simulink model "MotorCtrl_FOC_Physic"  (R2023b)
settings: Solver=FixedStepDiscrete  StartTime=0.0  StopTime=10  FixedStep=MC_Sim_BaseStep  RelTol=1e-3  EnableMultiTasking=on
values from neighbouring files (symbols this model uses):
  MC_MOS_DeadTime = 1.0E-6    [MotorControlDataDictionary_Math.sldd]    (also in MotorControlDataDictionary_Physic.sldd)
  MC_Motor_Mechinal_Inertia = 0.0103    [MotorControlDataDictionary_Math.sldd]    (also in MotorControlDataDictionary_Physic.sldd)
  MC_Motor_Phi = 0.0059190254913385806    [MotorControlDataDictionary_Math.sldd]    (also in MotorControlDataDictionary_Physic.sldd)
  MC_Motor_Rotor_Pn = 4.0    [MotorControlDataDictionary_Math.sldd]    (also in MotorControlDataDictionary_Physic.sldd)
  MC_Motor_Stator_Ld = 5.6345E-5    [MotorControlDataDictionary_Math.sldd]    (also in MotorControlDataDictionary_Physic.sldd)
  MC_Motor_Stator_Lq = 5.6345E-5    [MotorControlDataDictionary_Math.sldd]    (also in MotorControlDataDictionary_Physic.sldd)
  MC_Motor_Stator_Rs = 0.0286    [MotorControlDataDictionary_Math.sldd]    (also in MotorControlDataDictionary_Physic.sldd)
  MC_Param_CurrentPI_Ki = 0.0071879639914134473    [MotorControlDataDictionary_Math.sldd]    (also in MotorControlDataDictionary_Physic.sldd)
  MC_Param_CurrentPI_Kp = 0.283220860906427    [MotorControlDataDictionary_Math.sldd]    (also in MotorControlDataDictionary_Physic.sldd)
  MC_Param_CurrentPI_UdInteMax = 7.794228634059948    [MotorControlDataDictionary_Math.sldd]    (also in MotorControlDataDictionary_Physic.sldd)
  MC_Param_CurrentPI_UdInteMin = -7.794228634059948    [MotorControlDataDictionary_Math.sldd]    (also in MotorControlDataDictionary_Physic.sldd)
  MC_Param_CurrentPI_UdMax = 7.794228634059948    [MotorControlDataDictionary_Math.sldd]    (also in MotorControlDataDictionary_Physic.sldd)
  MC_Param_CurrentPI_UdMin = -7.794228634059948    [MotorControlDataDictionary_Math.sldd]    (also in MotorControlDataDictionary_Physic.sldd)
  MC_Param_CurrentPI_UqInteMax = 7.794228634059948    [MotorControlDataDictionary_Math.sldd]    (also in MotorControlDataDictionary_Physic.sldd)
  MC_Param_CurrentPI_UqInteMin = -7.794228634059948    [MotorControlDataDictionary_Math.sldd]    (also in MotorControlDataDictionary_Physic.sldd)
  MC_Param_CurrentPI_UqMax = 7.794228634059948    [MotorControlDataDictionary_Math.sldd]    (also in MotorControlDataDictionary_Physic.sldd)
  MC_Param_CurrentPI_UqMin = -7.794228634059948    [MotorControlDataDictionary_Math.sldd]    (also in MotorControlDataDictionary_Physic.sldd)
  MC_Param_Flux_Gamma = 750000.0    [MotorControlDataDictionary_Math.sldd]    (also in MotorControlDataDictionary_Physic.sldd)
  MC_Param_PhasetoReal = 500.0    [MotorControlDataDictionary_Math.sldd]    (also in MotorControlDataDictionary_Physic.sldd)
  MC_Param_SMO_CoffA = 0.97462064069571386    [MotorControlDataDictionary_Math.sldd]    (also in MotorControlDataDictionary_Physic.sldd)
  MC_Param_SMO_CoffB = 0.88739018546454884    [MotorControlDataDictionary_Math.sldd]    (also in MotorControlDataDictionary_Physic.sldd)
  MC_Param_SpeedCtrl_IdMax = 60.0    [MotorControlDataDictionary_Math.sldd]    (also in MotorControlDataDictionary_Physic.sldd)
  MC_Param_SpeedCtrl_IdMin = -60.0    [MotorControlDataDictionary_Math.sldd]    (also in MotorControlDataDictionary_Physic.sldd)
  MC_Param_SpeedCtrl_IqMax = 60.0    [MotorControlDataDictionary_Math.sldd]    (also in MotorControlDataDictionary_Physic.sldd)
  MC_Param_SpeedCtrl_IqMin = -60.0    [MotorControlDataDictionary_Math.sldd]    (also in MotorControlDataDictionary_Physic.sldd)
  MC_Param_SpeedPI_Ki = 0.57248683633241571    [MotorControlDataDictionary_Math.sldd]    (also in MotorControlDataDictionary_Physic.sldd)
  MC_Param_SpeedPI_Kp = 9.1114109857344836    [MotorControlDataDictionary_Math.sldd]    (also in MotorControlDataDictionary_Physic.sldd)
  MC_Param_SpeedtoTheta = 5.0E-5    [MotorControlDataDictionary_Math.sldd]    (also in MotorControlDataDictionary_Physic.sldd)
  MC_Param_SVPWM_DutyMax = 0.98    [MotorControlDataDictionary_Math.sldd]    (also in MotorControlDataDictionary_Physic.sldd)
  MC_Param_SVPWM_DutyMin = 0.02    [MotorControlDataDictionary_Math.sldd]    (also in MotorControlDataDictionary_Physic.sldd)
  MC_Param_SVPWM_SampleOffset1 = 0.02    [MotorControlDataDictionary_Math.sldd]    (also in MotorControlDataDictionary_Physic.sldd)
  MC_Param_SVPWM_SampleOffset2 = 0.015    [MotorControlDataDictionary_Math.sldd]    (also in MotorControlDataDictionary_Physic.sldd)
  MC_Param_SVPWM_SampleValid = 0.011999999999999999    [MotorControlDataDictionary_Math.sldd]    (also in MotorControlDataDictionary_Physic.sldd)
  MC_Sample_CurrentNoise = 1.0E-15    [MotorControlDataDictionary_Math.sldd]    (also in MotorControlDataDictionary_Physic.sldd)
  MC_Sample_VbusNoise = 1.0E-15    [MotorControlDataDictionary_Math.sldd]    (also in MotorControlDataDictionary_Physic.sldd)
  MC_Sim_BaseStep = 5.0E-8    [MotorControlDataDictionary_Math.sldd]    (also in MotorControlDataDictionary_Physic.sldd)
  MC_Sim_HFTStep = 5.0E-5    [MotorControlDataDictionary_Math.sldd]    (also in MotorControlDataDictionary_Physic.sldd)
  MC_Sim_MFTStep = 0.002    [MotorControlDataDictionary_Math.sldd]    (also in MotorControlDataDictionary_Physic.sldd)
libraries: simulink x17, nesl_utility x15, ee_lib x10, fl_lib x8
(part 1 of 3)
settings Model: DataDictionary=MotorControlDataDictionary_Physic.sldd  SimulationMode=accelerator  Creator=YXuan  LastModifiedBy=YXuan
settings SolverCC: AutoInsertRateTranBlk=on
settings OptimizationCC: DefaultParameterBehavior=Inlined  DefaultUnderspecifiedDataType=single  EnhancedBackFolding=on  PassReuseOutputArgsAs=Individual arguments  ZeroExternalMemoryAtStartup=off  ZeroInternalMemoryAtStartup=off  EfficientFloat2IntCast=on  OptimizeBlockOrder=speed  DifferentSizesBufferReuse=on  OptimizationCustomize=off  EfficientTunableParamExpr=on
settings DebuggingCC: ParameterPrecisionLossMsg=none
settings HardwareCC: ProdBitPerPointer=32  ProdBitPerSizeT=32  ProdBitPerPtrDiffT=32  ProdLargestAtomicInteger=Long  ProdLargestAtomicFloat=Double  ProdWordSize=32  ProdHWDeviceType=ARM Compatible->ARM Cortex-M
settings ModelReferenceCC: EnableRefExpFcnMdlSchedulingChecks=on
settings SFSimCC: MATLABDynamicMemAlloc=off
settings RTWCC: Description=Embedded Coder  SystemTargetFile=ert.tlc  GenCodeOnly=on  TemplateMakefile=ert_default_tmf  Toolchain=Microsoft Visual C++ 2022 v17.0 | nmake (64-bit Windows)
settings CodeAppCC: ForceParamTrailComments=on  IgnoreCustomStorageClasses=off  IgnoreTestpoints=on  OperatorAnnotations=on  SimulinkDataObjDesc=on  SFDataObjDesc=on  InsertBlockDesc=on
settings ERTTargetCC: TargetLangStandard=C99 (ISO)  InferredTypesCompatibility=on  GenerateSampleERTMain=on  CombineSignalStateStructs=on  SupportAbsoluteTime=off  SupportNonFinite=off  SupportComplex=off  RemoveDisableFunc=on  InlinedParameterPlacement=NonHierarchical  ERTCustomFileTemplate=example_file_process.tlc

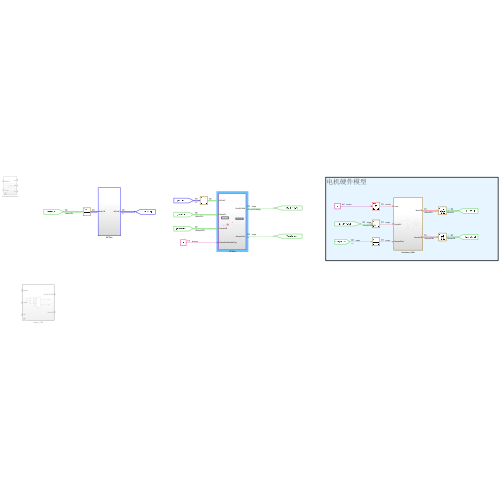
[thumbnail: Simulink's stored preview of the top-level diagram]
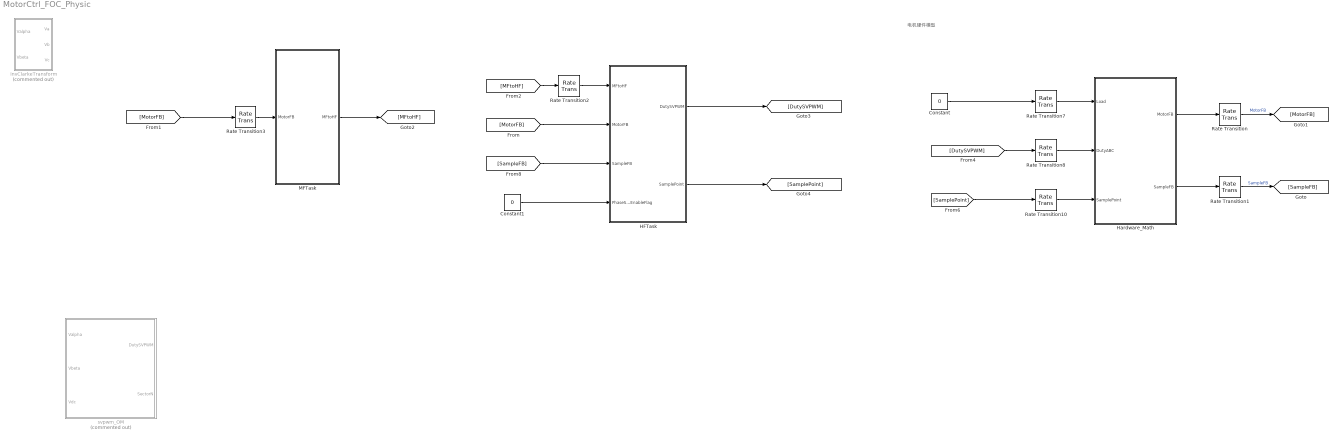
== system MotorCtrl_FOC_Physic ==
  note: 电机硬件模型
  Constant : Constant  Value=0
  Constant1 : Constant  Value=0  OutDataTypeStr=boolean
  HFTask : Subsystem  TreatAsAtomicUnit=on  SystemSampleTime=MC_Sim_HFTStep
  Hardware_Math : Subsystem  SystemSampleTime=MC_Sim_BaseStep  VariantControl=MC_Hardware_Motor_Model ==1&MC_Hardware_MotorMOS_Model==1
  MFTask : Subsystem  TreatAsAtomicUnit=on  SystemSampleTime=MC_Sim_MFTStep
  Rate Transition : RateTransition  OutPortSampleTime=MC_Sim_HFTStep
  Rate Transition1 : RateTransition  OutPortSampleTime=MC_Sim_HFTStep
  Rate Transition10 : RateTransition  OutPortSampleTime=MC_Sim_BaseStep
  Rate Transition2 : RateTransition  OutPortSampleTime=MC_Sim_HFTStep
  Rate Transition3 : RateTransition  OutPortSampleTime=MC_Sim_MFTStep
  Rate Transition7 : RateTransition  OutPortSampleTime=MC_Sim_BaseStep
  Rate Transition8 : RateTransition  OutPortSampleTime=MC_Sim_BaseStep
  invClarkeTransform : Subsystem  Commented=on
  svpwm_OM : Subsystem  Commented=on  TreatAsAtomicUnit=on  SystemSampleTime=MC_Sim_HFTStep
      settings: RTWSystemCode=Nonreusable function  RTWFcnNameOpts=Use subsystem name
  wires:
  Hardware_Math/2(SampleFB) -> Rate Transition1/1
  Rate Transition8/1 -> Hardware_Math/2(DutyABC)
  Hardware_Math/1(MotorFB) -> Rate Transition/1
  [SamplePoint] -> Rate Transition10/1
  [DutySVPWM] -> Rate Transition8/1
  Rate Transition1/1 -> [SampleFB]  "SampleFB"
  Constant/1 -> Rate Transition7/1
  Rate Transition10/1 -> Hardware_Math/3(SamplePoint)
  Rate Transition7/1 -> Hardware_Math/1(Load)
  Rate Transition/1 -> [MotorFB]  "MotorFB"
  HFTask/2(SamplePoint) -> [SamplePoint]
  Rate Transition2/1 -> HFTask/1(MFtoHF)
  [MFtoHF] -> Rate Transition2/1
  Rate Transition3/1 -> MFTask/1(MotorFB)
  Constant1/1 -> HFTask/4(PhaseShortEnableFlag)
  [MotorFB] -> Rate Transition3/1
  [SampleFB] -> HFTask/3(SampleFB)
  MFTask/1(MFtoHF) -> [MFtoHF]
  [MotorFB] -> HFTask/2(MotorFB)
  HFTask/1(DutySVPWM) -> [DutySVPWM]

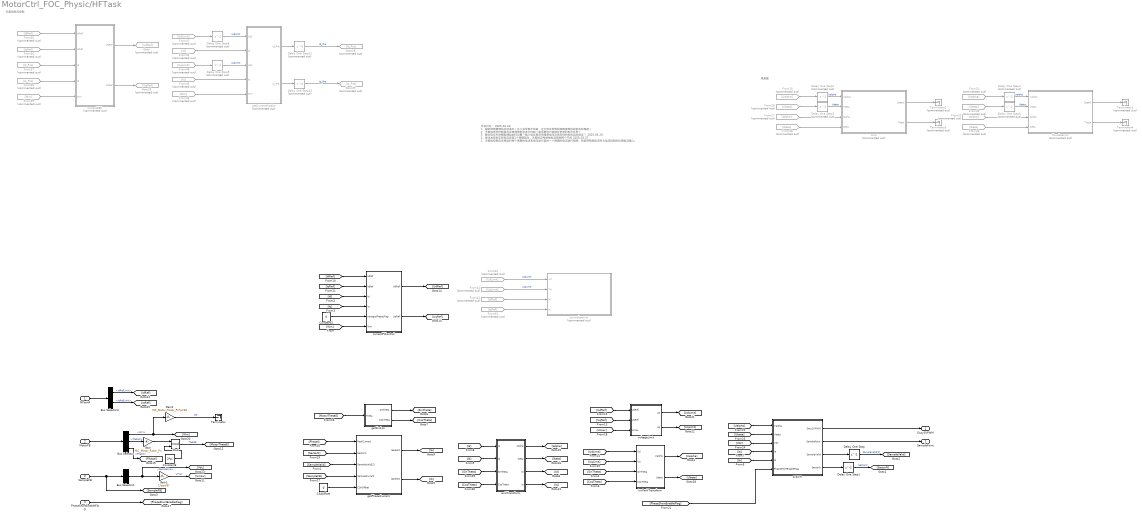
== system MotorCtrl_FOC_Physic/HFTask ==
  note: 观测器
  note: 无差拍电流控制
  note: 开发日志：
      | 2025.03.24:
      | 1、磁链观测器增益应该适中（过小会导致不收敛，过大则会导致观测角度相位超前实际角度）
      | 2、无差拍电流控制是否采用预测电流进行控制？是否要进行旋转反电势的电压补偿？
      | 3、静态电压补偿模型增益如何设置？输入电压是采用理想电压还是采样的电机实际电压？
      | 2025.03.25:
      | 1、测试发现电压和电流呈现2个周期延时，无差拍应考虑做电流预测两个节拍
      | 2025.03.27：
      | 1、无差拍控制应采用延时两个周期的电流和电压进行延时一个周期的电流进行预测，然后用预测电流作为电流控制的反馈电流输入。
  MFtoHF : Inport
  MotorFB : Inport  Port=2
  SampleFB : Inport  Port=3
  PhaseShortEnableFlag : Inport  Port=4
  Bus Selector : BusSelector  OutputSignals=Wm,ThetaM,PhaseI
  Bus Selector1 : BusSelector  OutputSignals=SampleVus
  Bus Selector3 : BusSelector  OutputSignals=IdRefLimit,IqRefLimit
  CSAOffset : Constant  Value=0  OutDataTypeStr=single
  Constant2 : Constant  Value=0  OutDataTypeStr=boolean
  Constant6 : Constant  Value=2*pi  OutDataTypeStr=single
  Delay One Step : Delay
  Delay One Step1 : Delay
  Delay One Step12 : Delay  Commented=on  DelayLength=0
  Delay One Step13 : Delay  Commented=on  DelayLength=0
  Delay One Step{2..5} (4 alike) : Delay  Commented=on
  Delay One Step8 : Delay  Commented=on  DelayLength=1
  Delay One Step9 : Delay  Commented=on  DelayLength=1
  From25 : From  Commented=on  GotoTag=Ualpha
  From26 : From  Commented=on  GotoTag=Ubeta
  From27 : From  Commented=on  GotoTag=Ialpha
  From28 : From  Commented=on  GotoTag=Ibeta
  From31 : From  Commented=on  GotoTag=Ualpha
  From32 : From  Commented=on  GotoTag=Ubeta
  From33 : From  Commented=on  GotoTag=Ialpha
  From34 : From  Commented=on  GotoTag=Ibeta
  From35 : From  Commented=on  GotoTag=IdRef
  From36 : From  Commented=on  GotoTag=IqRef
  From37 : From  Commented=on  GotoTag=Id_Pre
  From38 : From  Commented=on  GotoTag=Iq_Pre
  From39 : From  Commented=on  GotoTag=Wm
  From40 : From  Commented=on  GotoTag=UdLimit
  From41 : From  Commented=on  GotoTag=UqLimit
  From42 : From  Commented=on  GotoTag=IdRef
  From43 : From  Commented=on  GotoTag=IqRef
  From44 : From  Commented=on  GotoTag=Id
  From45 : From  Commented=on  GotoTag=Iq
  From46 : From  Commented=on  GotoTag=Wm
  From47 : From  Commented=on  GotoTag=UdLimit
  From48 : From  Commented=on  GotoTag=UqLimit
  Gain : Gain  Gain=MC_Motor_Rotor_Pn  OutDataTypeStr=single
  Gain1 : Gain  Gain=1/sqrt(3)  OutDataTypeStr=single
  Gain2 : Gain  Gain=MC_Motor_Rotor_Pn*pi/30
  Goto : Goto  Commented=on  GotoTag=UdRef
  Goto26 : Goto  Commented=on  GotoTag=UqRef
  Goto28 : Goto  Commented=on  GotoTag=Id_Pre
  Goto29 : Goto  Commented=on  GotoTag=Iq_Pre
  Mod : Math  Operator=mod
  Terminator : Terminator
  Terminator{1..4} (4 alike) : Terminator  Commented=on
  axisTransform : Subsystem
  currentDBC : Subsystem  Commented=on
  currentPIControl : Subsystem
  fluxobservor : Subsystem  Commented=on
  getCurrentPredict : Subsystem  Commented=on
  getPhaseCurrent : Subsystem
  getSinCos : Subsystem
  invParkTransform : Subsystem
  scvmobservor : Subsystem  Commented=on
  smo : Subsystem  Commented=on
  svpwm : Subsystem  TreatAsAtomicUnit=on
  voltageLimit : Subsystem
  DutySVPWM : Outport
  SamplePoint : Outport  Port=2
  wires:
  MFtoHF/1 -> Bus Selector3/1
  Delay One Step2/1 -> smo/1(Valpha)  "Ualpha"
  From25/1 -> Delay One Step2/1
  Delay One Step3/1 -> smo/2(Vbeta)  "Ubeta"
  From26/1 -> Delay One Step3/1
  From27/1 -> smo/3(Ialpha)
  From28/1 -> smo/4(Ibeta)
  smo/1(Speed) -> Terminator2/1
  smo/2(Theta) -> Terminator3/1
  [PhaseShortEnableFlag] -> svpwm/6(PhaseShortEnableFlag)
  [Umax] -> voltageLimit/3(Umax)
  svpwm/4(SectorN) -> Delay One Step1/1
  axisTransform/2(Ibeta) -> [Ibeta]
  svpwm/3(SampleValid) -> Delay One Step/1
  svpwm/1(DutySVPWM) -> DutySVPWM/1
  [SampleFB] -> getPhaseCurrent/4(SampleCurrent)
  [SectorN] -> getPhaseCurrent/2(SectorN)
  [UdRef] -> voltageLimit/1(UdRef)
  [UdLimit] -> invParkTransform/1(Ud)
  currentPIControl/1(UdRef) -> [UdRef]
  [Ubeta] -> svpwm/2(Vbeta)
  axisTransform/1(Ialpha) -> [Ialpha]
  [UqRef] -> voltageLimit/2(UqRef)
  [Ualpha] -> svpwm/1(Valpha)
  [Ia] -> axisTransform/1(Ia)
  svpwm/2(SamplePoint) -> SamplePoint/1
  currentPIControl/2(UqRef) -> [UqRef]
  [Vdc] -> svpwm/3(Vdc)
  voltageLimit/1(Ud) -> [UdLimit]
  [MotorThetaE] -> getSinCos/1(Theta)
  [Id] -> currentPIControl/3(Id)
  getSinCos/1(SinTheta) -> [SinTheta]
  [SampleValid] -> getPhaseCurrent/3(SampleValid[2])
  axisTransform/3(Id) -> [Id]
  getPhaseCurrent/2(Ibselect) -> [Ib]
  [Wm] -> currentPIControl/6(Wm)
  axisTransform/4(Iq) -> [Iq]
  [Iq] -> currentPIControl/4(Iq)
  Constant2/1 -> currentPIControl/5(IntregralResetFlag)
  [Ib] -> axisTransform/2(Ib)
  [UqLimit] -> invParkTransform/2(Uq)
  [SinTheta] -> invParkTransform/3(SinTheta)
  Delay One Step1/1 -> [SectorN]  "SectorN"
  [CosTheta] -> invParkTransform/4(CosTheta)
  [PhaseI] -> getPhaseCurrent/1(RealCurrent)
  invParkTransform/1(Ualpha) -> [Ualpha]
  Delay One Step/1 -> [SampleValid]  "SampleValid[2]"
  getSinCos/2(CosTheta) -> [CosTheta]
  voltageLimit/2(Uq) -> [UqLimit]
  [SinTheta] -> axisTransform/3(SinTheta)
  getPhaseCurrent/1(Iaselect) -> [Ia]
  CSAOffset/1 -> getPhaseCurrent/5(CSAOffset)
  [CosTheta] -> axisTransform/4(CosTheta)
  invParkTransform/2(Ubeta) -> [Ubeta]
  [Ib] -> svpwm/5(Ib)
  [Ia] -> svpwm/4(Ia)
  Bus Selector/2 -> Gain/1  "<ThetaM>"
  PhaseShortEnableFlag/1 -> [PhaseShortEnableFlag]
  Bus Selector/1 -> Gain2/1, [Wm]  "<Wm>"
  Mod/1 -> [MotorThetaE]  "ThetaE"
  Bus Selector/3 -> [PhaseI]  "<PhaseI>"
  Gain/1 -> Mod/1
  Bus Selector1/1 -> [Vdc], Gain1/1  "<SampleVus>"
  SampleFB/1 -> [SampleFB], Bus Selector1/1
  Gain1/1 -> [Umax]  "Umax"
  Constant6/1 -> Mod/2
  MotorFB/1 -> Bus Selector/1
  Bus Selector3/1 -> [IdRef]  "<IdRefLimit>"
  Bus Selector3/2 -> [IqRef]  "<IqRefLimit>"
  [IdRef] -> currentPIControl/1(IdRef)
  [IqRef] -> currentPIControl/2(IqRef)
  From34/1 -> fluxobservor/4(Ibeta)
  From33/1 -> fluxobservor/3(Ialpha)
  From32/1 -> Delay One Step5/1
  From31/1 -> Delay One Step4/1
  Delay One Step4/1 -> fluxobservor/1(Valpha)  "Ualpha"
  Delay One Step5/1 -> fluxobservor/2(Vbeta)  "Ubeta"
  fluxobservor/1(Speed) -> Terminator1/1
  fluxobservor/2(Theta) -> Terminator4/1
  currentDBC/2(UqRef) -> Goto26/1
  From36/1 -> currentDBC/2(IqRef)
  From35/1 -> currentDBC/1(IdRef)
  From37/1 -> currentDBC/3(Id)
  From38/1 -> currentDBC/4(Iq)
  From39/1 -> currentDBC/5(Wm)
  From41/1 -> scvmobservor/2(Vq)  "UqLimit"
  From40/1 -> scvmobservor/1(Vd)  "UdLimit"
  From42/1 -> scvmobservor/3(Id)
  From43/1 -> scvmobservor/4(Iq)
  Gain2/1 -> Terminator/1  "We"
  From44/1 -> getCurrentPredict/2(Id)
  From45/1 -> getCurrentPredict/4(Iq)
  From46/1 -> getCurrentPredict/5(Wm)
  From47/1 -> Delay One Step8/1
  From48/1 -> Delay One Step9/1
  getCurrentPredict/1(Id_Pre) -> Delay One Step12/1
  getCurrentPredict/2(Iq_Pre) -> Delay One Step13/1
  currentDBC/1(UdRef) -> Goto/1
  Delay One Step8/1 -> getCurrentPredict/1(Ud1)  "UdLimit"
  Delay One Step9/1 -> getCurrentPredict/3(Uq1)  "UqLimit"
  Delay One Step12/1 -> Goto28/1  "Id_Pre"
  Delay One Step13/1 -> Goto29/1  "Iq_Pre"

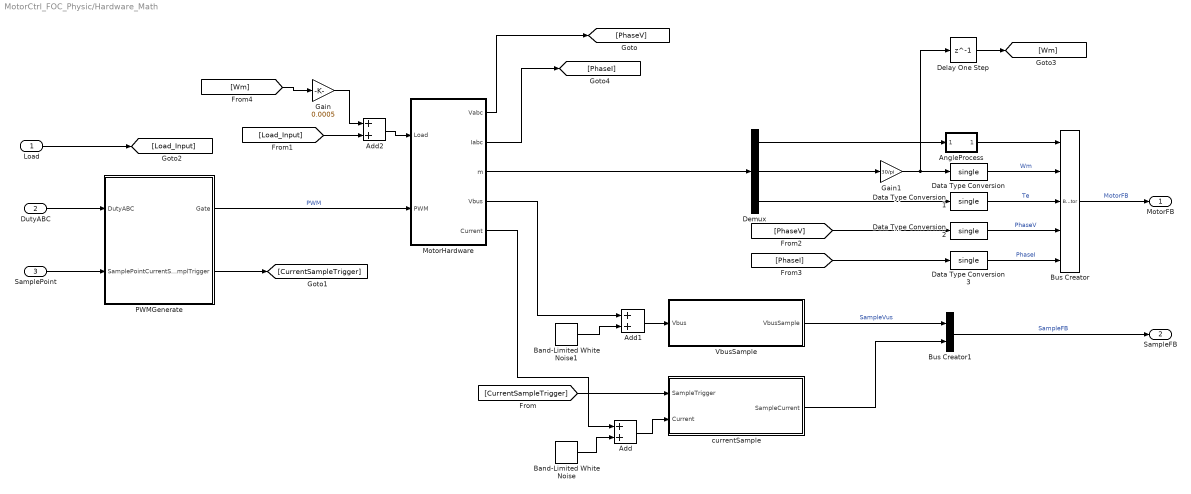
== system MotorCtrl_FOC_Physic/Hardware_Math ==
  Load : Inport
  DutyABC : Inport  Port=2
  SamplePoint : Inport  Port=3
  Add : Sum
  Add1 : Sum
  Add2 : Sum
  AngleProcess : Subsystem
  Band-Limited White Noise : simulink/Sources/Band-Limited White Noise  Cov=[MC_Sample_CurrentNoise]  Ts=MC_Sim_BaseStep  seed=[23341]
  Band-Limited White Noise1 : simulink/Sources/Band-Limited White Noise  Cov=[MC_Sample_VbusNoise]  Ts=MC_Sim_BaseStep  seed=[23341]
  Bus Creator : BusCreator  Inputs=5
  Bus Creator1 : BusCreator  Inputs=2
  Data Type Conversion{,1..3} (4 alike) : DataTypeConversion  OutDataTypeStr=single  SaturateOnIntegerOverflow=off  RndMeth=Floor
  Delay One Step : Delay  DelayLength=1
  Demux : Demux  Outputs=3
  Gain : Gain  Gain=0.0005
  Gain1 : Gain  Gain=30/pi
  MotorHardware : Subsystem
  PWMGenerate : Subsystem  SystemSampleTime=MC_Sim_BaseStep
  VbusSample : Subsystem
  currentSample : Subsystem  Variant=on  VariantControl=Subsystem
  MotorFB : Outport
  SampleFB : Outport  Port=2
  wires:
  Band-Limited White Noise/1 -> Add/2
  Add/1 -> currentSample/2(Current)
  Add1/1 -> VbusSample/1(Vbus)
  Band-Limited White Noise1/1 -> Add1/2
  [CurrentSampleTrigger] -> currentSample/1(SampleTrigger)
  PWMGenerate/2(CurrentSamplTrigger) -> [CurrentSampleTrigger]
  Demux/2 -> Gain1/1
  DutyABC/1 -> PWMGenerate/1(DutyABC)
  Demux/1 -> AngleProcess/1(In1)
  SamplePoint/1 -> PWMGenerate/2(SamplePoint)
  Demux/3 -> Data Type Conversion1/1
  Load/1 -> [Load_Input]
  Gain1/1 -> Delay One Step/1, Data Type Conversion/1
  AngleProcess/1(Out1) -> Bus Creator/1
  [PhaseV] -> Data Type Conversion2/1
  [PhaseI] -> Data Type Conversion3/1
  VbusSample/1(VbusSample) -> Bus Creator1/1  "SampleVus"
  currentSample/1(SampleCurrent) -> Bus Creator1/2
  Bus Creator1/1 -> SampleFB/1  "SampleFB"
  PWMGenerate/1(Gate) -> MotorHardware/2(PWM)  "PWM"
  MotorHardware/1(Vabc) -> [PhaseV]
  MotorHardware/2(Iabc) -> [PhaseI]
  MotorHardware/3(m) -> Demux/1
  MotorHardware/5(Current) -> Add/1
  MotorHardware/4(Vbus) -> Add1/1
  Data Type Conversion/1 -> Bus Creator/2  "Wm"
  Data Type Conversion1/1 -> Bus Creator/3  "Te"
  Data Type Conversion2/1 -> Bus Creator/4  "PhaseV"
  Data Type Conversion3/1 -> Bus Creator/5  "PhaseI"
  Bus Creator/1 -> MotorFB/1  "MotorFB"
  Add2/1 -> MotorHardware/1(Load)
  [Load_Input] -> Add2/2
  [Wm] -> Gain/1
  Gain/1 -> Add2/1
  Delay One Step/1 -> [Wm]

== system MotorCtrl_FOC_Physic/MFTask ==
  MotorFB : Inport
  Bus Creator : BusCreator  Inputs=2
  Bus Selector : BusSelector  OutputSignals=Wm
  Constant : Constant  Value=1500  OutDataTypeStr=single
  From2 : From  Commented=on  GotoTag=SpeedTarget
  From3 : From  Commented=on  GotoTag=SpeedMotor
  Goto : Goto  Commented=on  GotoTag=IdRef
  Goto1 : Goto  Commented=on  GotoTag=IqRef
  getCurrentLimit : Subsystem
  piofSpeed : Subsystem
  smcofSpeed : Subsystem  Commented=on
  MFtoHF : Outport
  wires:
  MotorFB/1 -> Bus Selector/1
  Bus Selector/1 -> [SpeedMotor]  "<Wm>"
  Bus Creator/1 -> MFtoHF/1
  smcofSpeed/1(IdRef) -> Goto/1
  smcofSpeed/2(IqRef) -> Goto1/1
  piofSpeed/1(IdRef) -> [IdRef]
  piofSpeed/2(IqRef) -> [IqRef]
  getCurrentLimit/2(IqRefLimit) -> [IqRefLimit]
  getCurrentLimit/1(IdRefLimit) -> [IdRefLimit]
  [IdRefLimit] -> Bus Creator/1
  [IqRefLimit] -> Bus Creator/2
  Constant/1 -> [SpeedTarget]  "SpeedTarget"
  From2/1 -> smcofSpeed/1(SpeedTarget)
  From3/1 -> smcofSpeed/2(SpeedReal)
  [IdRef] -> getCurrentLimit/1(IdRef)
  [IqRef] -> getCurrentLimit/2(IqRef)
  [SpeedTarget] -> piofSpeed/1(SpeedTarget)
  [SpeedMotor] -> piofSpeed/2(SpeedReal)

== system MotorCtrl_FOC_Physic/invClarkeTransform ==
  Valpha : Inport
  Vbeta : Inport  Port=2
  Add : Sum
  Gain : Gain  Gain=-1/2
  Gain1 : Gain  Gain=sqrt(3)/2
  Subtract : Sum  Inputs=+-
  Va : Outport
  Vb : Outport  Port=2
  Vc : Outport  Port=3
  wires:
  Valpha/1 -> Gain/1, Va/1  "Va"
  Vbeta/1 -> Gain1/1
  Gain/1 -> Subtract/1, Add/1
  Gain1/1 -> Subtract/2, Add/2
  Add/1 -> Vb/1  "Vb"
  Subtract/1 -> Vc/1  "Vc"

== system MotorCtrl_FOC_Physic/svpwm_OM ==
  Valpha : Inport
  Vbeta : Inport  Port=2
  Vdc : Inport  Port=3
  getVoltageExchange : Subsystem
  setDTCompelte : Subsystem
  DutySVPWM : Outport
  SectorN : Outport  Port=2
  wires:
  getVoltageExchange/4(Vmed) -> setDTCompelte/4(Vmed)
  getVoltageExchange/3(Vc) -> setDTCompelte/3(Vc)
  getVoltageExchange/2(Vb) -> setDTCompelte/2(Vb)
  getVoltageExchange/1(Va) -> setDTCompelte/1(Va)
  Vdc/1 -> getVoltageExchange/3(Vdc)
  Vbeta/1 -> getVoltageExchange/2(Vbeta)
  Valpha/1 -> getVoltageExchange/1(Valpha)
  setDTCompelte/2(DutyABC) -> DutySVPWM/1
  setDTCompelte/1(SectorN) -> SectorN/1

== system MotorCtrl_FOC_Physic/HFTask/axisTransform ==
  Ia : Inport
  Ib : Inport  Port=2
  SinTheta : Inport  Port=3
  CosTheta : Inport  Port=4
  Add1 : Sum
  Product{,1..3} (4 alike) : Product
  Signal Copy : SignalConversion  OverrideOpt=off
  Subtract : Sum  Inputs=-+
  a_plus_2b : Sum  Inputs=+++  RndMeth=Simplest  OutDataTypeStr=Inherit: Same as first input
  one_by_sqrt3 : Gain  Gain=1/sqrt(3)  RndMeth=Simplest  OutDataTypeStr=Inherit: Same as input
  Ialpha : Outport
  Ibeta : Outport  Port=2
  Id : Outport  Port=3
  Iq : Outport  Port=4
  wires:
  Product3/1 -> Subtract/2
  Product2/1 -> Subtract/1
  Add1/1 -> Id/1  "Id"
  Subtract/1 -> Iq/1  "Iq"
  Product/1 -> Add1/1
  Product1/1 -> Add1/2
  CosTheta/1 -> Product3/2, Product/2
  SinTheta/1 -> Product2/2, Product1/2
  a_plus_2b/1 -> one_by_sqrt3/1
  one_by_sqrt3/1 -> Ibeta/1, Product3/1, Product1/1  "Ibeta"
  Signal Copy/1 -> Ialpha/1, Product2/1, Product/1  "Ialpha"
  Ia/1 -> a_plus_2b/1, Signal Copy/1
  Ib/1 -> a_plus_2b/3, a_plus_2b/2

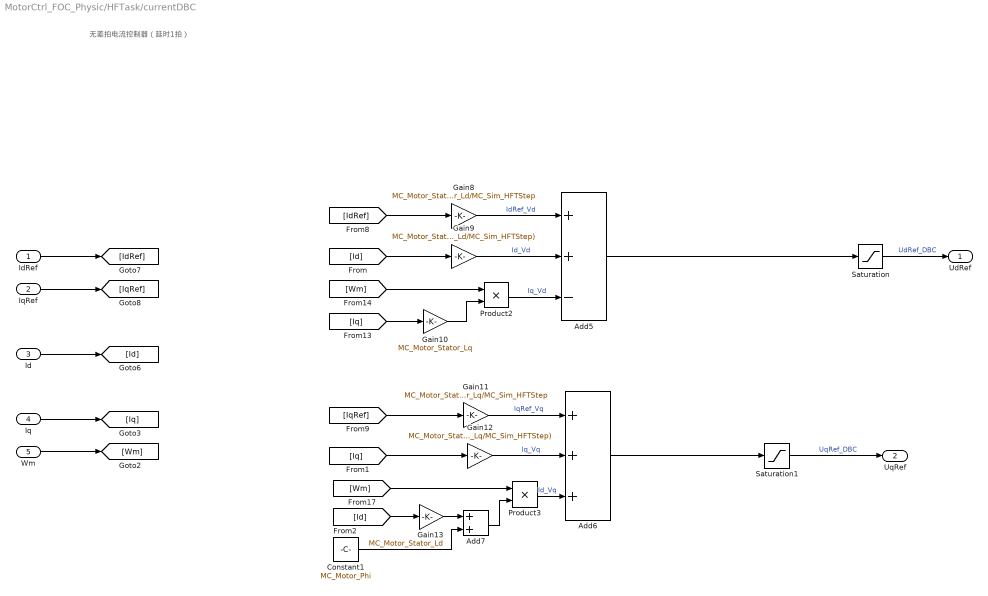
== system MotorCtrl_FOC_Physic/HFTask/currentDBC ==
  note: 无差拍电流控制器（延时1拍）
  IdRef : Inport
  IqRef : Inport  Port=2
  Id : Inport  Port=3
  Iq : Inport  Port=4
  Wm : Inport  Port=5
  Add5 : Sum  Inputs=++-
  Add6 : Sum  Inputs=+++
  Add7 : Sum
  Constant1 : Constant  Value=MC_Motor_Phi  OutDataTypeStr=single
  Gain10 : Gain  Gain=MC_Motor_Stator_Lq
  Gain11 : Gain  Gain=MC_Motor_Stator_Lq/MC_Sim_HFTStep
  Gain12 : Gain  Gain=MC_Motor_Stator_Rs-(MC_Motor_Stator_Lq/MC_Sim_HFTStep)
  Gain13 : Gain  Gain=MC_Motor_Stator_Ld
  Gain8 : Gain  Gain=MC_Motor_Stator_Ld/MC_Sim_HFTStep
  Gain9 : Gain  Gain=MC_Motor_Stator_Rs-(MC_Motor_Stator_Ld/MC_Sim_HFTStep)
  Product2 : Product
  Product3 : Product
  Saturation : Saturate  UpperLimit=MC_Param_CurrentPI_UdMax  LowerLimit=MC_Param_CurrentPI_UdMin
  Saturation1 : Saturate  UpperLimit=MC_Param_CurrentPI_UqMax  LowerLimit=MC_Param_CurrentPI_UqMin
  UdRef : Outport
  UqRef : Outport  Port=2
  wires:
  Wm/1 -> [Wm]
  Iq/1 -> [Iq]
  Id/1 -> [Id]
  IqRef/1 -> [IqRef]
  IdRef/1 -> [IdRef]
  [IdRef] -> Gain8/1
  Gain8/1 -> Add5/1  "IdRef_Vd"
  [Id] -> Gain9/1
  Gain9/1 -> Add5/2  "Id_Vd"
  [Iq] -> Gain10/1
  Gain10/1 -> Product2/2
  [Wm] -> Product2/1
  [IqRef] -> Gain11/1
  Gain11/1 -> Add6/1  "IqRef_Vq"
  Gain12/1 -> Add6/2  "Iq_Vq"
  [Iq] -> Gain12/1
  [Wm] -> Product3/1
  Add7/1 -> Product3/2
  Constant1/1 -> Add7/2
  Gain13/1 -> Add7/1
  [Id] -> Gain13/1
  Saturation/1 -> UdRef/1  "UdRef_DBC"
  Saturation1/1 -> UqRef/1  "UqRef_DBC"
  Add5/1 -> Saturation/1
  Product2/1 -> Add5/3  "Iq_Vd"
  Add6/1 -> Saturation1/1
  Product3/1 -> Add6/3  "Id_Vq"

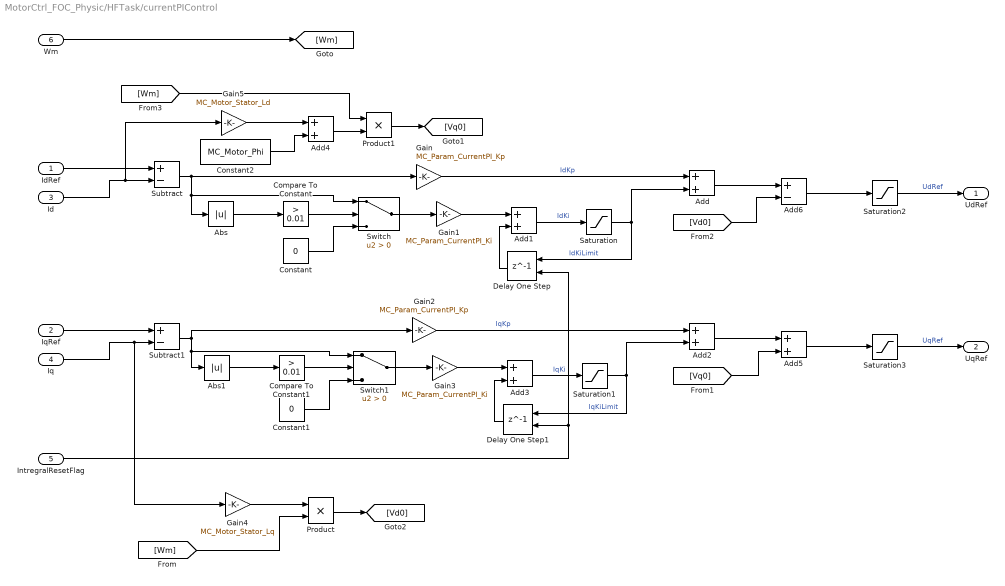
== system MotorCtrl_FOC_Physic/HFTask/currentPIControl ==
  IdRef : Inport
  IqRef : Inport  Port=2
  Id : Inport  Port=3
  Iq : Inport  Port=4
  IntregralResetFlag : Inport  Port=5
  Wm : Inport  Port=6
  Abs : Abs  SaturateOnIntegerOverflow=off
  Abs1 : Abs  SaturateOnIntegerOverflow=off
  Add{,2,4..5} (4 alike) : Sum
  Add1 : Sum  OutDataTypeStr=single
  Add3 : Sum  OutDataTypeStr=single
  Add6 : Sum  Inputs=+-
  Compare To Constant : simulink/Logic and Bit Operations/Compare To Constant  relop=>  const=0.01  OutDataTypeStr=boolean
  Compare To Constant1 : simulink/Logic and Bit Operations/Compare To Constant  relop=>  const=0.01  OutDataTypeStr=boolean
  Constant : Constant  Value=0  OutDataTypeStr=single
  Constant1 : Constant  Value=0  OutDataTypeStr=single
  Constant2 : Constant  Value=MC_Motor_Phi  OutDataTypeStr=single
  Delay One Step : Delay  DelayLength=1  ExternalReset=Level
      settings: InputPortMap=u0,r5
  Delay One Step1 : Delay  DelayLength=1  ExternalReset=Level
      settings: InputPortMap=u0,r5
  Gain : Gain  Gain=MC_Param_CurrentPI_Kp  OutDataTypeStr=single
  Gain1 : Gain  Gain=MC_Param_CurrentPI_Ki  OutDataTypeStr=single
  Gain2 : Gain  Gain=MC_Param_CurrentPI_Kp  OutDataTypeStr=single
  Gain3 : Gain  Gain=MC_Param_CurrentPI_Ki  OutDataTypeStr=single
  Gain4 : Gain  Gain=MC_Motor_Stator_Lq
  Gain5 : Gain  Gain=MC_Motor_Stator_Ld
  Product : Product
  Product1 : Product
  Saturation : Saturate  UpperLimit=MC_Param_CurrentPI_UdInteMax  LowerLimit=MC_Param_CurrentPI_UdInteMin
  Saturation1 : Saturate  UpperLimit=MC_Param_CurrentPI_UqInteMax  LowerLimit=MC_Param_CurrentPI_UqInteMin
  Saturation2 : Saturate  UpperLimit=MC_Param_CurrentPI_UdMax  LowerLimit=MC_Param_CurrentPI_UdMin
  Saturation3 : Saturate  UpperLimit=MC_Param_CurrentPI_UqMax  LowerLimit=MC_Param_CurrentPI_UqMin
  Subtract : Sum  Inputs=+-
  Subtract1 : Sum  Inputs=+-
  Switch : Switch  Criteria=u2 > Threshold  SaturateOnIntegerOverflow=off  InputSameDT=off
  Switch1 : Switch  Criteria=u2 > Threshold  SaturateOnIntegerOverflow=off  InputSameDT=off
  UdRef : Outport
  UqRef : Outport  Port=2
  wires:
  IdRef/1 -> Subtract/1
  Subtract/1 -> Gain/1, Switch/1, Abs/1
  Gain/1 -> Add/1  "IdKp"
  Abs/1 -> Compare To Constant/1
  Gain1/1 -> Add1/1
  Delay One Step/1 -> Add1/2
  Add1/1 -> Saturation/1  "IdKi"
  Saturation/1 -> Add/2, Delay One Step/1  "IdKiLimit"
  Saturation1/1 -> Delay One Step1/1, Add2/2  "IqKiLimit"
  Add3/1 -> Saturation1/1  "IqKi"
  Delay One Step1/1 -> Add3/2
  Gain3/1 -> Add3/1
  Gain2/1 -> Add2/1  "IqKp"
  Subtract1/1 -> Switch1/1, Abs1/1, Gain2/1
  Iq/1 -> Gain4/1, Subtract1/2
  IqRef/1 -> Subtract1/1
  IntregralResetFlag/1 -> Delay One Step/2, Delay One Step1/2
  Add5/1 -> Saturation3/1
  Switch/1 -> Gain1/1
  Compare To Constant/1 -> Switch/2
  Constant/1 -> Switch/3
  Constant1/1 -> Switch1/3
  Compare To Constant1/1 -> Switch1/2
  Abs1/1 -> Compare To Constant1/1
  Switch1/1 -> Gain3/1
  Gain4/1 -> Product/1
  Id/1 -> Gain5/1, Subtract/2
  [Wm] -> Product/2
  Gain5/1 -> Add4/1
  Add4/1 -> Product1/2
  Constant2/1 -> Add4/2
  Product1/1 -> [Vq0]
  Product/1 -> [Vd0]
  Add2/1 -> Add5/1
  [Vq0] -> Add5/2
  Add/1 -> Add6/1
  Add6/1 -> Saturation2/1
  [Vd0] -> Add6/2
  Saturation2/1 -> UdRef/1  "UdRef"
  Saturation3/1 -> UqRef/1  "UqRef"
  [Wm] -> Product1/1
  Wm/1 -> [Wm]

== system MotorCtrl_FOC_Physic/HFTask/fluxobservor ==
  Valpha : Inport
  Vbeta : Inport  Port=2
  Ialpha : Inport  Port=3
  Ibeta : Inport  Port=4
  getFlux : Subsystem
  getSpeedandTheta : Subsystem
  Speed : Outport
  Theta : Outport  Port=2
  wires:
  getSpeedandTheta/2(Theta) -> Theta/1
  getSpeedandTheta/1(Speed) -> Speed/1
  getFlux/2(Phibeta) -> getSpeedandTheta/2(Phibeta)
  getFlux/1(Phialpha) -> getSpeedandTheta/1(Phialpha)
  Ibeta/1 -> getFlux/4(Ibeta)
  Ialpha/1 -> getFlux/3(Ialpha)
  Vbeta/1 -> getFlux/2(Vbeta)
  Valpha/1 -> getFlux/1(Valpha)

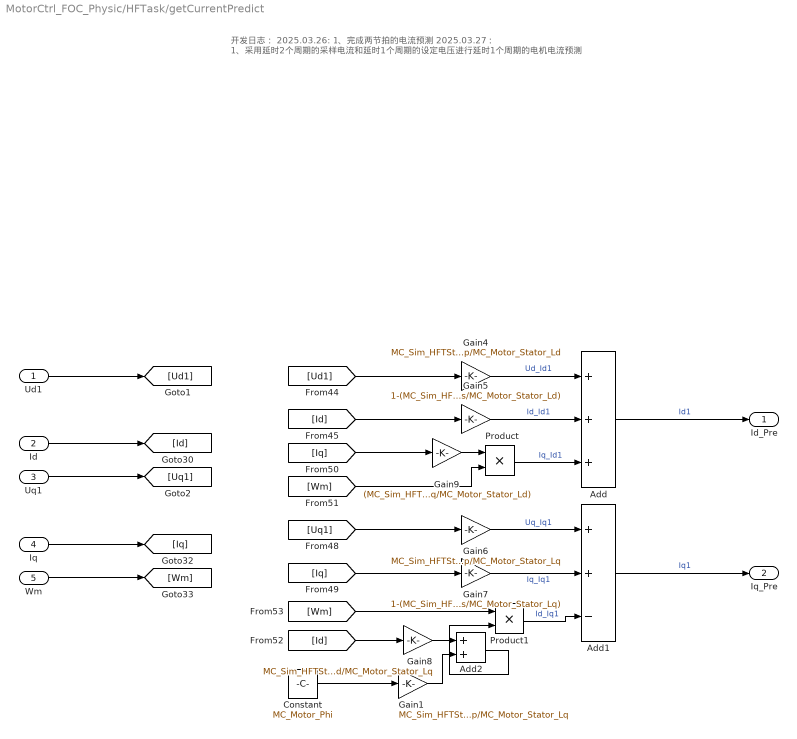
== system MotorCtrl_FOC_Physic/HFTask/getCurrentPredict ==
  note: 开发日志：
      | 2025.03.26:
      | 1、完成两节拍的电流预测
      | 2025.03.27：
      | 1、采用延时2个周期的采样电流和延时1个周期的设定电压进行延时1个周期的电机电流预测
  Ud1 : Inport
  Id : Inport  Port=2
  Uq1 : Inport  Port=3
  Iq : Inport  Port=4
  Wm : Inport  Port=5
  Add : Sum  Inputs=+++
  Add1 : Sum  Inputs=++-
  Add2 : Sum
  Constant : Constant  Value=MC_Motor_Phi  OutDataTypeStr=single
  Gain1 : Gain  Gain=MC_Sim_HFTStep/MC_Motor_Stator_Lq
  Gain4 : Gain  Gain=MC_Sim_HFTStep/MC_Motor_Stator_Ld
  Gain5 : Gain  Gain=1-(MC_Sim_HFTStep*MC_Motor_Stator_Rs/MC_Motor_Stator_Ld)
  Gain6 : Gain  Gain=MC_Sim_HFTStep/MC_Motor_Stator_Lq
  Gain7 : Gain  Gain=1-(MC_Sim_HFTStep*MC_Motor_Stator_Rs/MC_Motor_Stator_Lq)
  Gain8 : Gain  Gain=MC_Sim_HFTStep*MC_Motor_Stator_Ld/MC_Motor_Stator_Lq
  Gain9 : Gain  Gain=(MC_Sim_HFTStep*MC_Motor_Stator_Lq/MC_Motor_Stator_Ld)
  Product : Product
  Product1 : Product
  Id_Pre : Outport
  Iq_Pre : Outport  Port=2
  wires:
  [Iq] -> Gain7/1
  [Wm] -> Product1/1
  Iq/1 -> [Iq]
  Gain4/1 -> Add/1  "Ud_Id1"
  [Iq] -> Gain9/1
  [Uq1] -> Gain6/1
  Gain9/1 -> Product/1
  Constant/1 -> Gain1/1
  Product/1 -> Add/3  "Iq_Id1"
  [Ud1] -> Gain4/1
  Gain6/1 -> Add1/1  "Uq_Iq1"
  Gain7/1 -> Add1/2  "Iq_Iq1"
  Gain5/1 -> Add/2  "Id_Id1"
  [Id] -> Gain8/1
  Product1/1 -> Add1/3  "Id_Iq1"
  Gain8/1 -> Add2/1
  [Wm] -> Product/2
  Id/1 -> [Id]
  Add2/1 -> Product1/2
  [Id] -> Gain5/1
  Wm/1 -> [Wm]
  Gain1/1 -> Add2/2
  Add/1 -> Id_Pre/1  "Id1"
  Add1/1 -> Iq_Pre/1  "Iq1"
  Ud1/1 -> [Ud1]
  Uq1/1 -> [Uq1]

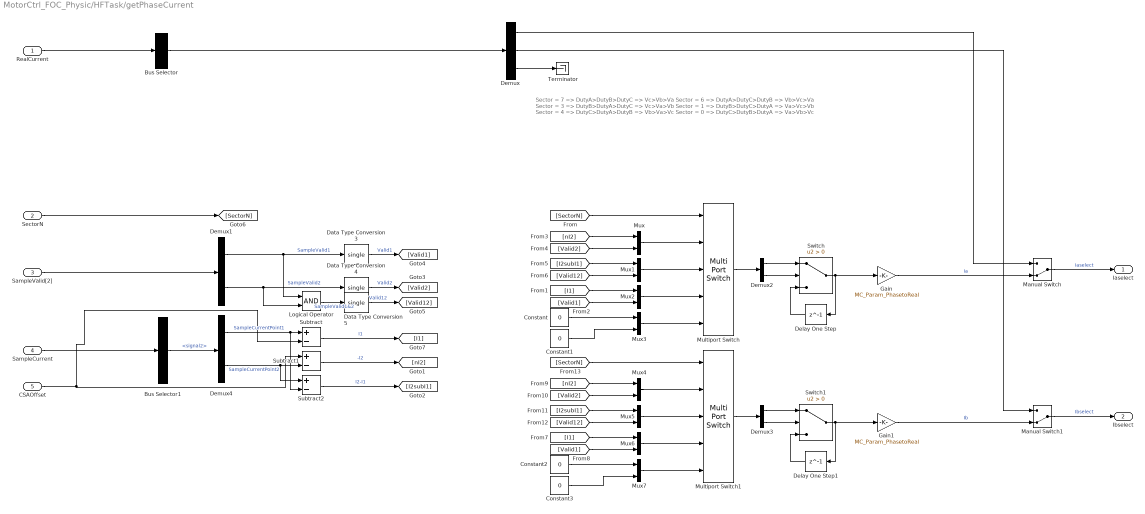
== system MotorCtrl_FOC_Physic/HFTask/getPhaseCurrent ==
  note: Sector = 7 => DutyA>DutyB>DutyC => Vc>Vb>Va
      | Sector = 6 => DutyA>DutyC>DutyB => Vb>Vc>Va
      | Sector = 3 => DutyB>DutyA>DutyC => Vc>Va>Vb
      | Sector = 1 => DutyB>DutyC>DutyA => Va>Vc>Vb
      | Sector = 4 => DutyC>DutyA>DutyB => Vb>Va>Vc
      | Sector = 0 => DutyC>DutyB>DutyA => Va>Vb>Vc
  RealCurrent : Inport
  SectorN : Inport  Port=2
  SampleValid[2] : Inport  Port=3
  SampleCurrent : Inport  Port=4
  CSAOffset : Inport  Port=5
  Bus Selector : BusSelector  OutputSignals=PhaseI  OutputAsBus=on
  Bus Selector1 : BusSelector  OutputSignals=signal2
  Constant{,1..3} (4 alike) : Constant  Value=0  OutDataTypeStr=single
  Data Type Conversion3 : DataTypeConversion  OutDataTypeStr=single  RndMeth=Simplest  SaturateOnIntegerOverflow=off
  Data Type Conversion4 : DataTypeConversion  OutDataTypeStr=single  RndMeth=Simplest  SaturateOnIntegerOverflow=off
  Data Type Conversion5 : DataTypeConversion  OutDataTypeStr=single  RndMeth=Simplest  SaturateOnIntegerOverflow=off
  Delay One Step : Delay  DelayLength=1
  Delay One Step1 : Delay  DelayLength=1
  Demux : Demux  Outputs=3
  Demux{1..4} (4 alike) : Demux  Outputs=2
  Gain : Gain  Gain=MC_Param_PhasetoReal
  Gain1 : Gain  Gain=MC_Param_PhasetoReal
  Logical Operator : Logic  AllPortsSameDT=off  OutDataTypeStr=boolean
  Manual Switch : ManualSwitch  CurrentSetting=0
  Manual Switch1 : ManualSwitch  CurrentSetting=0
  Multiport Switch : MultiPortSwitch  DataPortOrder=Specify indices  DataPortIndices={[7,6],[3,4],[0,1]}  DataPortForDefault=Additional data port  SaturateOnIntegerOverflow=off  InputSameDT=off
  Multiport Switch1 : MultiPortSwitch  DataPortOrder=Specify indices  DataPortIndices={[3,1],[7,0],[6,4]}  DataPortForDefault=Additional data port  SaturateOnIntegerOverflow=off  InputSameDT=off
  Mux{,1..7} (8 alike) : Mux  Inputs=2
  Subtract : Sum  Inputs=+-
  Subtract1 : Sum  Inputs=+-
  Subtract2 : Sum  Inputs=+-
  Switch : Switch  Criteria=u2 > Threshold  SaturateOnIntegerOverflow=off  InputSameDT=off
  Switch1 : Switch  Criteria=u2 > Threshold  SaturateOnIntegerOverflow=off  InputSameDT=off
  Terminator : Terminator
  Iaselect : Outport
  Ibselect : Outport  Port=2
  wires:
  RealCurrent/1 -> Bus Selector/1
  Bus Selector/1 -> Demux/1
  Manual Switch/1 -> Iaselect/1  "Iaselect"
  Demux/3 -> Terminator/1
  Manual Switch1/1 -> Ibselect/1  "Ibselect"
  Multiport Switch1/1 -> Demux3/1
  Demux3/2 -> Switch1/2
  Demux3/1 -> Switch1/1
  Switch1/1 -> Delay One Step1/1, Gain1/1
  Delay One Step1/1 -> Switch1/3
  Gain1/1 -> Manual Switch1/2  "Ib"
  Gain/1 -> Manual Switch/2  "Ia"
  Delay One Step/1 -> Switch/3
  Switch/1 -> Gain/1, Delay One Step/1
  Demux2/1 -> Switch/1
  Demux2/2 -> Switch/2
  Multiport Switch/1 -> Demux2/1
  [SectorN] -> Multiport Switch1/1
  Mux4/1 -> Multiport Switch1/2
  Mux5/1 -> Multiport Switch1/3
  Mux6/1 -> Multiport Switch1/4
  [I1] -> Mux6/1
  [Valid1] -> Mux6/2
  [nI2] -> Mux4/1
  [Valid2] -> Mux4/2
  [Valid12] -> Mux5/2
  [I2subI1] -> Mux5/1
  Mux7/1 -> Multiport Switch1/5
  Constant2/1 -> Mux7/1
  Constant3/1 -> Mux7/2
  Subtract/1 -> [I1]  "I1"
  Subtract1/1 -> [nI2]  "-I2"
  Data Type Conversion5/1 -> [Valid12]  "Valid12"
  Data Type Conversion4/1 -> [Valid2]  "Valid2"
  Data Type Conversion3/1 -> [Valid1]  "Valid1"
  Subtract2/1 -> [I2subI1]  "I2-I1"
  Constant1/1 -> Mux3/2
  Constant/1 -> Mux3/1
  Mux3/1 -> Multiport Switch/5
  [I2subI1] -> Mux1/1
  [Valid12] -> Mux1/2
  [Valid2] -> Mux/2
  [nI2] -> Mux/1
  [Valid1] -> Mux2/2
  [I1] -> Mux2/1
  [SectorN] -> Multiport Switch/1
  SectorN/1 -> [SectorN]
  Mux2/1 -> Multiport Switch/4
  Mux1/1 -> Multiport Switch/3
  Mux/1 -> Multiport Switch/2
  Logical Operator/1 -> Data Type Conversion5/1  "SampleValid1&2"
  Demux1/2 -> Data Type Conversion4/1, Logical Operator/2  "SampleValid2"
  Demux1/1 -> Data Type Conversion3/1, Logical Operator/1  "SampleValid1"
  SampleValid[2]/1 -> Demux1/1
  Demux4/2 -> Subtract2/1, Subtract1/2  "SampleCurrentPoint2"
  CSAOffset/1 -> Subtract1/1, Subtract/2
  Demux4/1 -> Subtract2/2, Subtract/1  "SampleCurrentPoint1"
  Bus Selector1/1 -> Demux4/1  "<signal2>"
  SampleCurrent/1 -> Bus Selector1/1
  Demux/1 -> Manual Switch/1
  Demux/2 -> Manual Switch1/1

== system MotorCtrl_FOC_Physic/HFTask/getSinCos ==
  Theta : Inport
  Sin : Trigonometry
  Sin1 : Trigonometry  Operator=cos
  SinTheta : Outport
  CosTheta : Outport  Port=2
  wires:
  Theta/1 -> Sin1/1, Sin/1
  Sin/1 -> SinTheta/1
  Sin1/1 -> CosTheta/1

== system MotorCtrl_FOC_Physic/HFTask/invParkTransform ==
  Ud : Inport
  Uq : Inport  Port=2
  SinTheta : Inport  Port=3
  CosTheta : Inport  Port=4
  Add : Sum
  Product{,1..3} (4 alike) : Product
  Subtract : Sum  Inputs=+-
  Ualpha : Outport
  Ubeta : Outport  Port=2
  wires:
  Uq/1 -> Product3/1, Product1/1
  Subtract/1 -> Ualpha/1  "Ualpha"
  CosTheta/1 -> Product/2, Product3/2
  SinTheta/1 -> Product2/2, Product1/2
  Product/1 -> Subtract/1
  Product1/1 -> Subtract/2
  Ud/1 -> Product/1, Product2/1
  Product2/1 -> Add/1
  Product3/1 -> Add/2
  Add/1 -> Ubeta/1  "Ubeta"

== system MotorCtrl_FOC_Physic/HFTask/scvmobservor ==
  Vd : Inport
  Vq : Inport  Port=2
  Id : Inport  Port=3
  Iq : Inport  Port=4
  getW : Subsystem
  wires:
  Vd/1 -> getW/1(Vd)
  Vq/1 -> getW/2(Vq)
  Id/1 -> getW/3(Id)
  Iq/1 -> getW/4(Iq)

== system MotorCtrl_FOC_Physic/HFTask/smo ==
  Valpha : Inport
  Vbeta : Inport  Port=2
  Ialpha : Inport  Port=3
  Ibeta : Inport  Port=4
  getE : Subsystem
  getSpeedandTheta : Subsystem
  Speed : Outport
  Theta : Outport  Port=2
  wires:
  Valpha/1 -> getE/1(Valpha)
  Vbeta/1 -> getE/2(Vbeta)
  Ialpha/1 -> getE/3(Ialpha)
  Ibeta/1 -> getE/4(Ibeta)
  getE/1(Ealpha) -> getSpeedandTheta/1(Ealpha)
  getE/2(Ebeta) -> getSpeedandTheta/2(Ebeta)
  getSpeedandTheta/1(Speed) -> Speed/1
  getSpeedandTheta/2(Theta) -> Theta/1

== system MotorCtrl_FOC_Physic/HFTask/svpwm ==
  Valpha : Inport
  Vbeta : Inport  Port=2
  Vdc : Inport  Port=3
  Ia : Inport  Port=4
  Ib : Inport  Port=5
  PhaseShortEnableFlag : Inport  Port=6
  Terminator : Terminator
  getVoltageExchange : Subsystem
  setDTCompelte : Subsystem
  setPhaseandSample_ORS_Double : Subsystem
  DutySVPWM : Outport
  SamplePoint : Outport  Port=2
  SampleValid : Outport  Port=3
  SectorN : Outport  Port=4
  wires:
  Valpha/1 -> getVoltageExchange/1(Valpha)
  Vbeta/1 -> getVoltageExchange/2(Vbeta)
  Vdc/1 -> getVoltageExchange/3(Vdc)
  getVoltageExchange/1(Va) -> setDTCompelte/1(Va)
  getVoltageExchange/2(Vb) -> setDTCompelte/2(Vb)
  getVoltageExchange/3(Vc) -> setDTCompelte/3(Vc)
  getVoltageExchange/4(Vmed) -> setDTCompelte/4(Vmed)
  Ia/1 -> setDTCompelte/5(Ia)
  Ib/1 -> setDTCompelte/6(ib)
  setDTCompelte/1(SectorN) -> SectorN/1, setPhaseandSample_ORS_Double/1(SectorN)
  setDTCompelte/2(DutyLMS) -> setPhaseandSample_ORS_Double/2(DutyLMS)
  setPhaseandSample_ORS_Double/1(DutySVPWM) -> DutySVPWM/1
  setPhaseandSample_ORS_Double/2(SamplePoint) -> SamplePoint/1
  setPhaseandSample_ORS_Double/3(SampleValid) -> SampleValid/1
  PhaseShortEnableFlag/1 -> Terminator/1

== system MotorCtrl_FOC_Physic/HFTask/voltageLimit ==
  UdRef : Inport
  UqRef : Inport  Port=2
  Umax : Inport  Port=3
  Add : Sum
  Compare To Constant : simulink/Logic and Bit Operations/Compare To Constant  relop=<=  const=0  OutDataTypeStr=boolean
  Compare To Constant1 : simulink/Logic and Bit Operations/Compare To Constant  relop=>=  const=0  OutDataTypeStr=boolean
  Constant : Constant  Value=0  OutDataTypeStr=single
  Gain : Gain  Gain=-1
  Gain1 : Gain  Gain=-1
  Product : Product
  Saturation Dynamic : simulink/Discontinuities/Saturation Dynamic  OutMin=[]  OutMax=[]  OutDataTypeStr=Inherit: Same as second input  OutDataType=fixdt(1, 16)  OutScaling=2^-10  DoSatur=off
  Sqrt : Sqrt
  Subtract : Sum  Inputs=+-
  Switch : Switch  Criteria=u2 > Threshold  SaturateOnIntegerOverflow=off  InputSameDT=off
  Switch1 : Switch  Criteria=u2 > Threshold  SaturateOnIntegerOverflow=off  InputSameDT=off
  Switch2 : Switch  Criteria=u2 > Threshold  SaturateOnIntegerOverflow=off  InputSameDT=off
  Ud : Outport
  Uq : Outport  Port=2
  wires:
  Add/1 -> Product/1
  Subtract/1 -> Product/2
  Product/1 -> Compare To Constant/1, Sqrt/1
  Compare To Constant/1 -> [UdOverFlow]
  Sqrt/1 -> Gain/1, Saturation Dynamic/1
  Gain/1 -> Saturation Dynamic/3
  UdRef/1 -> [UdRef]
  UqRef/1 -> [UqRef]
  Umax/1 -> [Umax]
  [Umax] -> Subtract/1, Add/1
  [UdRef] -> Add/2, Subtract/2
  [UqRef] -> Saturation Dynamic/2
  Saturation Dynamic/1 -> Switch/3
  [UdOverFlow] -> Switch/2
  Constant/1 -> Switch/1
  Switch/1 -> Uq/1  "UqLimit"
  Switch1/1 -> Ud/1  "UdLimit"
  Switch2/1 -> Switch1/1
  [UdRef] -> Compare To Constant1/1
  Compare To Constant1/1 -> Switch2/2
  [Umax] -> Gain1/1, Switch2/1
  Gain1/1 -> Switch2/3
  [UdOverFlow] -> Switch1/2
  [UdRef] -> Switch1/3

== system MotorCtrl_FOC_Physic/Hardware_Math/AngleProcess ==
  In1 : Inport
  Constant : Constant  Value=2*pi  SampleTime=-1
  Data Type Conversion : DataTypeConversion  OutDataTypeStr=single  SaturateOnIntegerOverflow=off  RndMeth=Floor
  Mod : Math  Operator=mod
  Out1 : Outport
  wires:
  Mod/1 -> Data Type Conversion/1
  In1/1 -> Mod/1
  Constant/1 -> Mod/2
  Data Type Conversion/1 -> Out1/1  "ThetaM"
